simulink model "TWIP_Balancing_Robot0"  (R2020a)
settings: Solver=ode23t  StartTime=0.0  StopTime=13  FixedStep=1e-3  MaxStep=0.01  RelTol=1e-4  AbsTol=1e-5  EnableMultiTasking=on
StartFcn:
  | tic;
StopFcn:
  | Elapsed_Sim_Time = toc;
  | disp(['Elapsed Sim Time = ' num2str(Elapsed_Sim_Time)]);
model workspace (MAT data in the model file):
  l_whl_trq = [0; 0; 0; 0.00025; 0; 0; 0; -0.00025; 0.0005; 0; 0; 0; -0.0005; 0.00025; 0; 0; 0; -0.00025; -0.00075; 0; 0; 0; 0.00075]
  r_whl_trq = [0; 0; 0; 0.001; 0; 0; 0; -0.001; 0.0005; 0; 0; 0; -0.0005; 0.0005; 0; 0; 0; -0.0005; -0.00075; 0; 0; 0; 0.00075]
  table.length = 1
  table.thickness = 0.01
  tableWhl.contact.k = 1000
  tableWhl.contact.b = 100
  whl.rad = 0.025
  whl.thickness = 0.005
settings Model: Creator=smiller  LastModifiedBy=User
settings SolverCC: AutoScaleAbsTol=off
settings DataIOCC: MaxDataPoints=15000  SaveFormat=Array  SaveOutput=off  SaveTime=off  ReturnWorkspaceOutputs=off  SignalLoggingName=logsout_Robot_2_Whl
settings OptimizationCC: LifeSpan=inf
settings DebuggingCC: SolverPrmCheckMsg=warning  UnconnectedInputMsg=none  UnconnectedOutputMsg=none  AllowSymbolicDim=off  PregeneratedLibrarySubsystemCodeDiagnostic=none  SFUnexpectedBacktrackingDiag=warning  SFNoUnconditionalDefaultTransitionDiag=warning  SFExecutionAtInitializationDiag=none  ArithmeticOperatorsInVariantConditions=warning
settings HardwareCC: ProdBitPerPointer=32  ProdBitPerSizeT=32  ProdBitPerPtrDiffT=32  ProdLargestAtomicFloat=None  ProdIntDivRoundTo=Undefined  ProdEndianess=Unspecified  ProdWordSize=32  ProdHWDeviceType=32-bit Generic
settings ModelReferenceCC: PropagateSignalLabelsOutOfModel=off
settings SFSimCC: SimUseLocalCustomCode=off  CustomCodeUndefinedFunction=UseInterfaceOnly
settings RTWCC: RTWUseLocalCustomCode=off
settings CodeAppCC: StateflowObjectComments=on
settings GRTTargetCC: TargetLangStandard=C89/C90 (ANSI)
settings ConfigComp: CovMetricSettings=dw  CovHtmlReporting=on  CovSaveCumulativeToWorkspaceVar=on  CovSaveSingleToWorkspaceVar=on  CovExternalEMLEnable=off  CovSFcnEnable=off
settings SimscapeCC: SimscapeNormalizeSystem=off  SimscapeLogType=all  SimscapeLogSimulationStatistics=on  SimscapeLogName=simlog_Robot_2_Whl  SimscapeLogDataHistory=15000
settings ConfigurationSet: Description=SimMechanics 2G
settings DiagnosticsConfigSet: SimMechanicsRigidlyBoundBlock=none
settings ExplorerConfigSet: InternalSimMechanicsExplorerSettings="<ExplorerConfiguration><canonicalview>default</canonicalview><AnimationSetting><BasePlaybackSpeed>1.0</BasePlaybackSpeed><PlaybackSpeedFactor>4.0</PlaybackSpeedFactor></AnimationSetting><TilePanel><TileInfo><Tiles Columns=\"1\" Count=\"1\" Rows=\"1\"><Column Left=\"2\" Weight=\"1\"/><Column Left=\"524\"/><Row Top=\"2\" Weight=\"1\"/><Row Top=\"463\"/><Tile Height=\"1\" Width=\"1\" X=\"0\" Y=\"0\"/></Tiles></TileInfo><SceneInfo><SceneViewer><BGColor><R>0.91372549533843994</R><G>0.9529411792755127</G><B>0.9529411792755127</B></BGColor><Camera><Position><X>-1.2788736799007898</X><Y>0.11117500897827101</Y><Z>0.74683506413493239</Z></Position><Center><X>0</X><Y>0</Y><Z>0.028405746445059776</Z></Center><Up><X>0.4897961701570378</X><Y>0.00030785872423301237</Y><Z>0.87183692105949728</Z></Up><Left>-0.55939182937145238</Left><Right>0.55939182937145238</Right><Bottom>-0.28958761096000674</Bottom><Top>0.28958761096000674</Top></Camera></SceneViewer></SceneInfo></TilePanel></ExplorerConfiguration>"

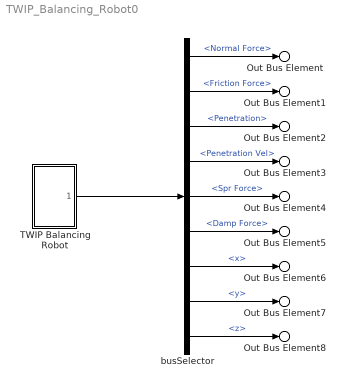
== system TWIP_Balancing_Robot0 ==
  TWIP Balancing Robot : Subsystem  TreatAsAtomicUnit=on  ReferencedSubsystem=TWIP_Balancing_Robot
  busSelector : BusSelector  OutputSignals=Normal Force,Friction Force,Penetration,Penetration Vel,Spr Force,Damp Force,Frame Sep.x,Frame Sep.y,Frame Sep.z
  Out Bus Element : Outport  PortName=Out1  Element=Normal Force
  Out Bus Element1 : Outport  PortName=Out1  Element=Friction Force
  Out Bus Element2 : Outport  PortName=Out1  Element=Penetration
  Out Bus Element3 : Outport  PortName=Out1  Element=Penetration Vel
  Out Bus Element4 : Outport  PortName=Out1  Element=Spr Force
  Out Bus Element5 : Outport  PortName=Out1  Element=Damp Force
  Out Bus Element6 : Outport  PortName=Out1  Element=Frame Sep.x
  Out Bus Element7 : Outport  PortName=Out1  Element=Frame Sep.y
  Out Bus Element8 : Outport  PortName=Out1  Element=Frame Sep.z
  wires:
  busSelector/9 -> Out Bus Element8/1  "<z>"
  busSelector/5 -> Out Bus Element4/1  "<Spr Force>"
  busSelector/1 -> Out Bus Element/1  "<Normal Force>"
  busSelector/6 -> Out Bus Element5/1  "<Damp Force>"
  busSelector/2 -> Out Bus Element1/1  "<Friction Force>"
  TWIP Balancing Robot/1 -> busSelector/1
  busSelector/7 -> Out Bus Element6/1  "<x>"
  busSelector/3 -> Out Bus Element2/1  "<Penetration>"
  busSelector/8 -> Out Bus Element7/1  "<y>"
  busSelector/4 -> Out Bus Element3/1  "<Penetration Vel>"
